simulink model "MdEnChk"  (R2018b)
settings: Solver=FixedStepDiscrete  StartTime=0.0  StopTime=10.0  FixedStep=0.01  RelTol=1e-3
undefined symbols (not defined in the file or in its folder): IsStBsy32_Set, ModeState32_Set, SetBit
settings Model: Creator=sn2xws  LastModifiedBy=sn2xws
settings DataIOCC: SaveFormat=StructureWithTime
settings OptimizationCC: DefaultParameterBehavior=Inlined  EnhancedBackFolding=on  PassReuseOutputArgsAs=Individual arguments  ZeroExternalMemoryAtStartup=off  ZeroInternalMemoryAtStartup=off  OptimizeBlockOrder=speed  DifferentSizesBufferReuse=on  OptimizationCustomize=off
settings DebuggingCC: ParameterTunabilityLossMsg=error
settings SFSimCC: MATLABDynamicMemAlloc=off
settings RTWCC: SystemTargetFile=autosar.tlc  GenCodeOnly=on  TemplateMakefile=ert_default_tmf  Description=AUTOSAR  GenerateReport=on  IncludeHyperlinkInReport=on  LaunchReport=on  GenerateTraceInfo=on  GenerateTraceReport=on  GenerateTraceReportSl=on  GenerateTraceReportSf=on  GenerateTraceReportEml=on  GenerateCodeMetricsReport=on
settings CodeAppCC: ForceParamTrailComments=on  IgnoreCustomStorageClasses=off  OperatorAnnotations=on  SimulinkDataObjDesc=on  SFDataObjDesc=on  InsertBlockDesc=on
settings STFCustomTargetCC: TargetLangStandard=C99 (ISO)  MultiwordLength=256  ParMdlRefBuildCompliant=on  CompOptLevelCompliant=on  IncludeMdlTerminateFcn=off  CombineOutputUpdateFcns=on  SuppressErrorStatus=on  ERTCustomFileBanners=on  SupportNonFinite=off  SupportComplex=off  SupportContinuousTime=off  SupportNonInlinedSFcns=off  RemoveResetFunc=on  MATLABClassNameForMDSCustomization=Simulink.SoftwareTarget.ERTCustomization  AutosarCompliant=on  UseToolchainInfoCompliant=on  LookupTableObjectStructAxisOrder=2,1,3,4,...  LUTObjectStructOrderEvenSpacing=Size,Table,Breakpoints  SystemTargetFile=autosar.tlc
settings ERTTargetCC: TargetLangStandard=C99 (ISO)  ConcurrentExecutionCompliant=off  IncludeMdlTerminateFcn=off  SuppressErrorStatus=on  SupportNonFinite=off  SupportComplex=off  ModelStepFunctionPrototypeControlCompliant=off  CPPClassGenCompliant=off  AutosarCompliant=on  LookupTableObjectStructAxisOrder=2,1,3,4,...  LUTObjectStructOrderEvenSpacing=Size,Table,Breakpoints  InlinedParameterPlacement=NonHierarchical  ERTCustomFileTemplate=example_file_process.tlc  ERTFilePackagingFormat=Compact

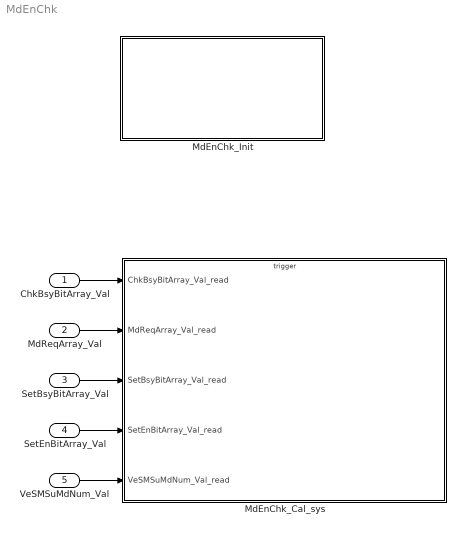
== system MdEnChk ==
  ChkBsyBitArray_Val : Inport  OutDataTypeStr=uint32  PortDimensions=32
  MdReqArray_Val : Inport  Port=2  OutDataTypeStr=boolean  PortDimensions=32
  SetBsyBitArray_Val : Inport  Port=3  OutDataTypeStr=uint32  PortDimensions=32
  SetEnBitArray_Val : Inport  Port=4  OutDataTypeStr=uint32  PortDimensions=32
  VeSMSuMdNum_Val : Inport  Port=5  OutDataTypeStr=uint8  PortDimensions=1
  MdEnChk_Cal_sys : Subsystem
  MdEnChk_Init : Subsystem
  wires:
  ChkBsyBitArray_Val/1 -> MdEnChk_Cal_sys/1(ChkBsyBitArray_Val_read)
  MdReqArray_Val/1 -> MdEnChk_Cal_sys/2(MdReqArray_Val_read)
  SetBsyBitArray_Val/1 -> MdEnChk_Cal_sys/3(SetBsyBitArray_Val_read)
  SetEnBitArray_Val/1 -> MdEnChk_Cal_sys/4(SetEnBitArray_Val_read)
  VeSMSuMdNum_Val/1 -> MdEnChk_Cal_sys/5(VeSMSuMdNum_Val_read)

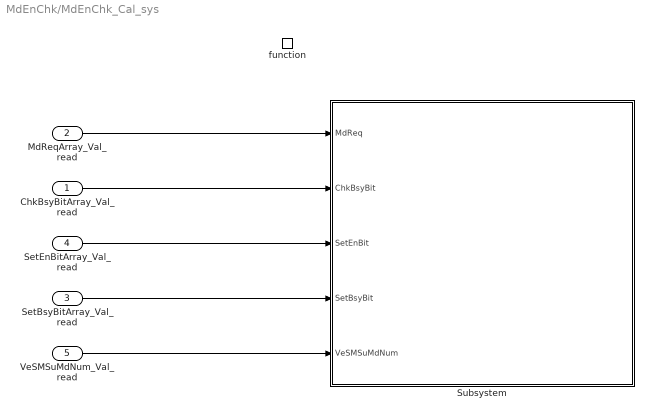
== system MdEnChk/MdEnChk_Cal_sys ==
  ChkBsyBitArray_Val_read : Inport
  MdReqArray_Val_read : Inport  Port=2
  SetBsyBitArray_Val_read : Inport  Port=3
  SetEnBitArray_Val_read : Inport  Port=4
  VeSMSuMdNum_Val_read : Inport  Port=5
  function : TriggerPort  TriggerType=function-call  IsSimulinkFunction=on  FunctionName=MdEnChk_Cal  VariantControl=(inherit)
  Subsystem : Subsystem
  wires:
  MdReqArray_Val_read/1 -> Subsystem/1(MdReq)
  ChkBsyBitArray_Val_read/1 -> Subsystem/2(ChkBsyBit)
  SetEnBitArray_Val_read/1 -> Subsystem/3(SetEnBit)
  VeSMSuMdNum_Val_read/1 -> Subsystem/5(VeSMSuMdNum)
  SetBsyBitArray_Val_read/1 -> Subsystem/4(SetBsyBit)

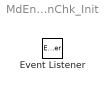
== system MdEnChk/MdEnChk_Init ==
  Event Listener : EventListener  EventName=reset

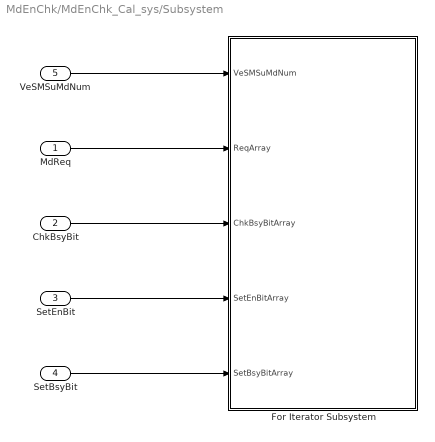
== system MdEnChk/MdEnChk_Cal_sys/Subsystem ==
  MdReq : Inport
  ChkBsyBit : Inport  Port=2
  SetEnBit : Inport  Port=3
  SetBsyBit : Inport  Port=4
  VeSMSuMdNum : Inport  Port=5
  For Iterator Subsystem : Subsystem  TreatAsAtomicUnit=on
  wires:
  MdReq/1 -> For Iterator Subsystem/2(ReqArray)
  ChkBsyBit/1 -> For Iterator Subsystem/3(ChkBsyBitArray)
  SetEnBit/1 -> For Iterator Subsystem/4(SetEnBitArray)
  SetBsyBit/1 -> For Iterator Subsystem/5(SetBsyBitArray)
  VeSMSuMdNum/1 -> For Iterator Subsystem/1(VeSMSuMdNum)

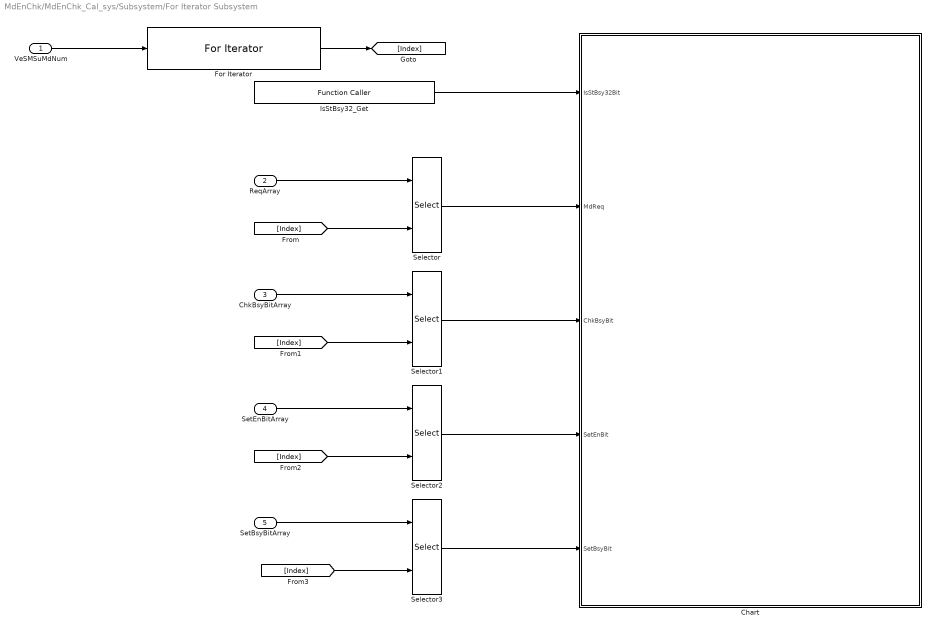
== system MdEnChk/MdEnChk_Cal_sys/Subsystem/For Iterator Subsystem ==
  VeSMSuMdNum : Inport
  ReqArray : Inport  Port=2
  ChkBsyBitArray : Inport  Port=3
  SetEnBitArray : Inport  Port=4
  SetBsyBitArray : Inport  Port=5
  Chart : Stateflow chart  TreatAsAtomicUnit=on
  For Iterator : ForIterator  IterationSource=external  IndexMode=Zero-based  IterationVariableDataType=int8
  IsStBsy32_Get : FunctionCaller  FunctionPrototype=IsStBsy32Bit = IsStBsy32_Get()  OutputArgumentSpecifications=uint32(1)
  Selector{,1..3} (4 alike) : Selector  IndexMode=Zero-based  InputPortWidth=32  IndexOptions=Index vector (port)  Indices=[1 3]  OutputSizes=1
  wires:
  VeSMSuMdNum/1 -> For Iterator/1
  SetBsyBitArray/1 -> Selector3/1
  Selector1/1 -> Chart/3(ChkBsyBit)
  Selector/1 -> Chart/2(MdReq)
  SetEnBitArray/1 -> Selector2/1
  [Index] -> Selector1/2
  ReqArray/1 -> Selector/1
  Selector2/1 -> Chart/4(SetEnBit)
  Selector3/1 -> Chart/5(SetBsyBit)
  [Index] -> Selector3/2
  [Index] -> Selector/2
  [Index] -> Selector2/2
  ChkBsyBitArray/1 -> Selector1/1
  For Iterator/1 -> [Index]
  IsStBsy32_Get/1 -> Chart/1(IsStBsy32Bit)

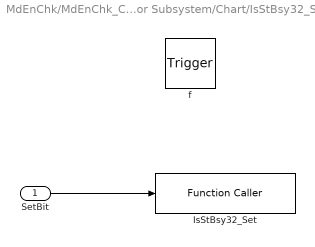
== system MdEnChk/MdEnChk_Cal_sys/Subsystem/For Iterator Subsystem/Chart/IsStBsy32_Set ==
  SetBit : Inport
  f : TriggerPort  TriggerType=function-call  VariantControl=(inherit)
      settings: CopyFcn=Stateflow.SLINSF.SimulinkMan.removeBlockPreDeleteFcn  PreDeleteFcn=Stateflow.SLINSF.SimulinkMan.unsafePredeleteFcn
  IsStBsy32_Set : FunctionCaller  FunctionPrototype=IsStBsy32_Set(SetBit)  InputArgumentSpecifications=uint32(1)
  wires:
  SetBit/1 -> IsStBsy32_Set/1

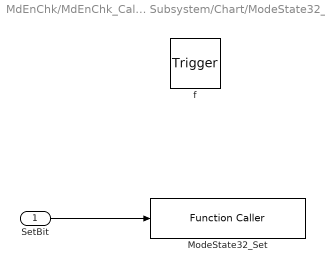
== system MdEnChk/MdEnChk_Cal_sys/Subsystem/For Iterator Subsystem/Chart/ModeState32_Set ==
  SetBit : Inport
  f : TriggerPort  TriggerType=function-call  VariantControl=(inherit)
      settings: CopyFcn=Stateflow.SLINSF.SimulinkMan.removeBlockPreDeleteFcn  PreDeleteFcn=Stateflow.SLINSF.SimulinkMan.unsafePredeleteFcn
  ModeState32_Set : FunctionCaller  FunctionPrototype=ModeState32_Set(SetBit)  InputArgumentSpecifications=uint32(1)
  wires:
  SetBit/1 -> ModeState32_Set/1

== stateflow chart MdEnChk/MdEnChk_Cal_sys/Subsystem/For Iterator Subsystem/Chart ==
  state IsStBsy32_Set(SetBit) [function]
  state ModeState32_Set(SetBit) [function]
  (default) -> (junction 252)
  (junction 252) -> (junction 249) [order 1] : [MdReq&&((IsStBsy32Bit&ChkBsyBit)==0)]
  (junction 252) -> (junction 251) [order 2]
  (junction 249) -> (junction 250) : {
      | ModeState32_Set(SetEnBit);
      | IsStBsy32_Set(SetBsyBit);
      | }
  (junction 250) -> (junction 251)
  (junction 251) -> (junction 258)
  data: SetBit function_input; SetBit function_input; IsStBsy32Bit input; MdReq input; ChkBsyBit input; SetEnBit input; SetBsyBit input
